simulink model "Controlador"  (R2015a)
settings: Solver=ode45  StartTime=0.0  StopTime=Tsim  RelTol=1e-4
settings Model: Creator=pedro  LastModifiedBy=Administrator
settings OptimizationCC: ExpressionDepthLimit=2147483647
settings DebuggingCC: UnderspecifiedInitializationDetection=Classic  MergeDetectMultiDrivingBlocksExec=none  SolverPrmCheckMsg=warning  StateNameClashWarn=warning

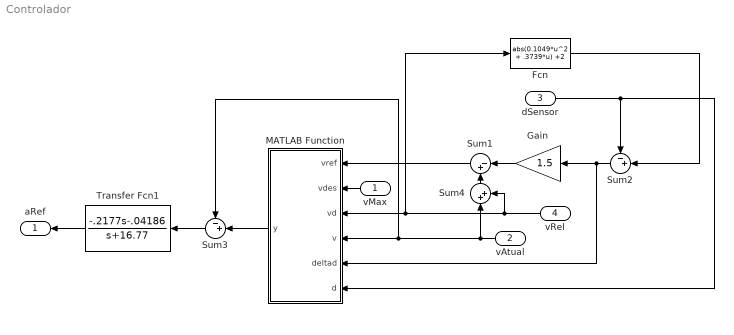
== system Controlador ==
  vMax : Inport
  vAtual : Inport  Port=2
  dSensor : Inport  Port=3
  vRel : Inport  Port=4
  Fcn : Fcn  Expr=abs(0.1049*u^2 + .3739*u) +2
  Gain : Gain  Gain=1.5
  MATLAB Function : MATLAB Function  TreatAsAtomicUnit=on
  Sum1 : Sum  Inputs=|-+
  Sum2 : Sum  Inputs=-+|
  Sum3 : Sum  Inputs=-+|
  Sum4 : Sum  Inputs=|++
  Transfer Fcn1 : TransferFcn  Numerator=[-.2177 -.04186]  Denominator=[1 16.77]
  aRef : Outport
  wires:
  dSensor/1 -> MATLAB Function/6(d), Sum2/1
  Sum2/1 -> MATLAB Function/5(deltad), Gain/1
  Gain/1 -> Sum1/1
  MATLAB Function/1(y) -> Sum3/2
  Sum1/1 -> MATLAB Function/1(vref)
  vMax/1 -> MATLAB Function/2(vdes)
  Sum3/1 -> Transfer Fcn1/1
  Transfer Fcn1/1 -> aRef/1
  Fcn/1 -> Sum2/2
  vAtual/1 -> Sum4/1, Sum3/1, MATLAB Function/4(v)
  vRel/1 -> Sum4/2, Fcn/1, MATLAB Function/3(vd)
  Sum4/1 -> Sum1/2

== matlab function Controlador/MATLAB Function ==
  data: vref input; vdes input; y output; vd input; v input; deltad input; d input
function y   = fcn(vref, vdes, vd, v, deltad,d)
%#codegen
%if(deltad<0)
%    y=vdes;
%end

%if(deltad>0 && v<vref)
%    y=vref;
%end


% if(deltad<0)
%     y=vdes;
% elseif(v<vref)
%     y=min(vdes, vref);
% elseif(vd<0)
%     y=min(vdes, vref);
% else
%     y=vdes;
% end

%if(d >=10)

    if(deltad<0)
        y=vdes;
    else
        if(v<vref)
            y=min(vdes, vref);
        else
            if(vd < 0)
                y=min(vdes, vref);
            else
                y = vdes;
            end
        end
    end
% else
%     y = 0;
%     flag = 0;
%end
